simulink model "ToyModel_sliding_friction"  (R2017a)
settings: Solver=ode45  StartTime=0.0  StopTime=T  RelTol=2.8421709430404007E-14  AbsTol=2.8421709430404007E-14
values from neighbouring files (symbols this model uses):
  f_s1 = 0    [Pointmass_circle_spacial_path.m]
  f_s2 = 0    [Pointmass_circle_spacial_path.m]
  g = 9.8    [Pointmass_circle_spacial_path.m]
  mass = 2    [Pointmass_circle_spacial_path.m]
  radius = 2    [Pointmass_circle_spacial_path.m]
  x1_0 = radius*cos(phase)    [Pointmass_circle_spacial_path.m]
  x2_0 = radius*sin(phase)    [Pointmass_circle_spacial_path.m]
settings Model: PauseTimes=0.1  NumberOfSteps=50  Creator=cc16g15  LastModifiedBy=cchoc
settings SolverCC: MaxConsecutiveMinStep=100  ZeroCrossAlgorithm=Adaptive
settings DebuggingCC: InheritedTsInSrcMsg=none

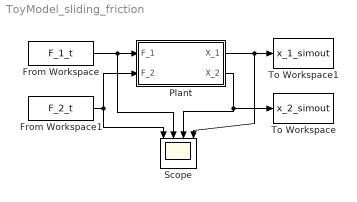
== system ToyModel_sliding_friction ==
  From Workspace : FromWorkspace  VariableName=F_1_t  OutDataTypeStr=double  OutputAfterFinalValue=Setting to zero
  From Workspace1 : FromWorkspace  VariableName=F_2_t  OutDataTypeStr=double  OutputAfterFinalValue=Setting to zero
  Plant : Subsystem
  Scope : Scope  NumInputPorts=4
  To Workspace : ToWorkspace  VariableName=x_2_simout  SaveFormat=Timeseries  SampleTime=-1
  To Workspace1 : ToWorkspace  VariableName=x_1_simout  SaveFormat=Timeseries  SampleTime=-1
  wires:
  From Workspace/1 -> Scope/2, Plant/1(F_1)
  From Workspace1/1 -> Scope/1, Plant/2(F_2)
  Plant/2(X_2) -> Scope/3, To Workspace/1
  Plant/1(X_1) -> To Workspace1/1, Scope/4

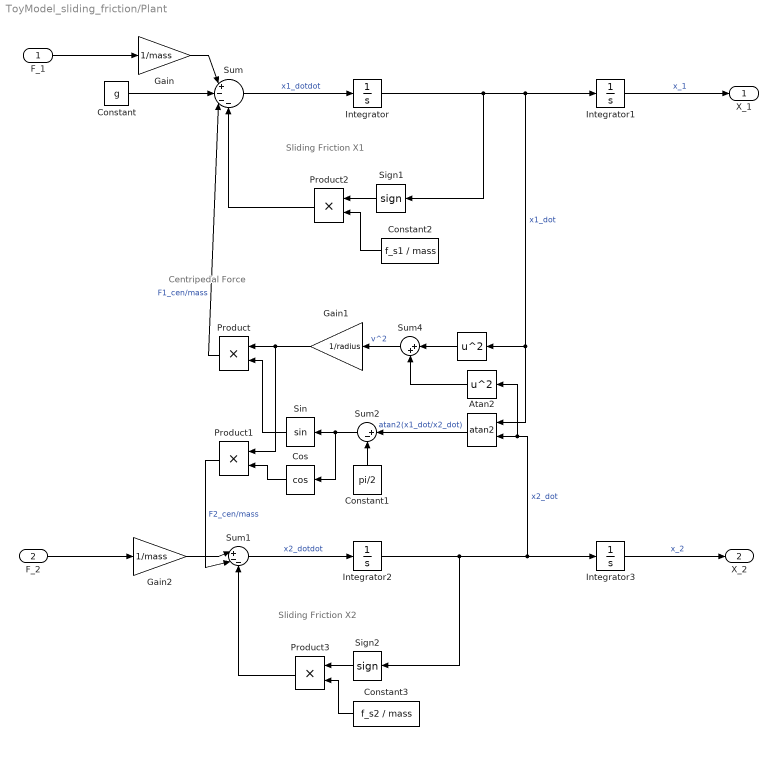
== system ToyModel_sliding_friction/Plant ==
  note: Centripedal Force
  note: Sliding Friction X2
  note: Sliding Friction X1
  F_1 : Inport
  F_2 : Inport  Port=2
  " " : Math  Operator=square  OutputSignalType=real
  " " : Math  Operator=square  OutputSignalType=real  SaturateOnIntegerOverflow=on
  Atan2 : Trigonometry  Operator=atan2
  Constant : Constant  Value=g
  Constant1 : Constant  Value=pi/2
  Constant2 : Constant  Value=f_s1 / mass
  Constant3 : Constant  Value=f_s2 / mass
  Cos : Trigonometry  Operator=cos
  Gain : Gain  Gain=1/mass
  Gain1 : Gain  Gain=1/radius
  Gain2 : Gain  Gain=1/mass
  Integrator : Integrator  ZeroCross=off
  Integrator1 : Integrator  InitialCondition=x1_0  ZeroCross=off
  Integrator2 : Integrator  ZeroCross=off
  Integrator3 : Integrator  InitialCondition=x2_0  ZeroCross=off
  Product{,1..3} (4 alike) : Product
  Sign1 : Signum  ZeroCross=off
  Sign2 : Signum  ZeroCross=off
  Sin : Trigonometry
  Sum : Sum  Inputs=|+---
  Sum1 : Sum  Inputs=|+--
  Sum2 : Sum  Inputs=|+-
  Sum4 : Sum  Inputs=|++
  X_1 : Outport
  X_2 : Outport  Port=2
  wires:
  Sum/1 -> Integrator/1  "x1_dotdot"
  Integrator/1 -> Sign1/1, Integrator1/1, " "/1, Atan2/1  "x1_dot"
  Sum1/1 -> Integrator2/1  "x2_dotdot"
  F_2/1 -> Gain2/1
  Integrator2/1 -> Integrator3/1, Atan2/2, " "/1, Sign2/1  "x2_dot"
  Integrator1/1 -> X_1/1  "x_1"
  Integrator3/1 -> X_2/1  "x_2"
  Gain2/1 -> Sum1/1
  " "/1 -> Sum4/1
  " "/1 -> Sum4/2
  Constant/1 -> Sum/2
  F_1/1 -> Gain/1
  Gain/1 -> Sum/1
  Sum4/1 -> Gain1/1  "v^2"
  Atan2/1 -> Sum2/1  "atan2(x1_dot/x2_dot)"
  Constant1/1 -> Sum2/2
  Product/1 -> Sum/3  "F1_cen/mass"
  Product1/1 -> Sum1/2  "F2_cen/mass"
  Gain1/1 -> Product1/1, Product/1
  Sum2/1 -> Cos/1, Sin/1
  Sin/1 -> Product/2
  Cos/1 -> Product1/2
  Sign1/1 -> Product2/1
  Sign2/1 -> Product3/1
  Constant2/1 -> Product2/2
  Product2/1 -> Sum/4
  Constant3/1 -> Product3/2
  Product3/1 -> Sum1/3
